simulink model "pneumatic04212025"  (R2024b)
settings: Solver=VariableStepAuto  StartTime=0.0  StopTime=20  RelTol=1e-3
values from neighbouring files (symbols this model uses):
  A1 = 3.1416e-04    (= 0.00031416)    [InitialParameter.m]    (also in pneumatic_code.m = 0.000314159265359)
  A2 = 2.6389e-04    (= 0.00026389)    [InitialParameter.m]    (also in pneumatic_code.m = 0.000263893782902)
  Ap = Ar    (= 5.02654824574e-05)    [pneumatic_code.m]
  b = 1    [InitialParameter.m]    (also in pneumatic_code.m = 0.0025)
  Beta = 50    [pneumatic_code.m]
  beta_s = 8*10^-3    (= 0.008)    [pneumatic_code.m]
  C1 = sqrt((k/R)*(2/(k+1))^((k+1)/(k-1)))    [pneumatic_code.m]
  C2 = sqrt((2*k)/(R*(k-1)))    [pneumatic_code.m]
  Cf = .25    (= 0.25)    [pneumatic_code.m]
  ep = 0.0024    [InitialParameter.m]    (also in pneumatic_code.m = 0.02)
  g1 = 9    [InitialParameter.m]    (also in pneumatic_code.m = 10)
  g2 = 4    [InitialParameter.m]    (also in pneumatic_code.m = 9)
  g3 = 18    [InitialParameter.m]    (also in pneumatic_code.m = 5)
  g4 = 0.32    [InitialParameter.m]    (also in pneumatic_code.m = 3)
  g5 = 3    [pneumatic_code.m]
  gamma1 = R*T*k    (= 118129.2)    [pneumatic_code.m]
  k = 1.4    [pneumatic_code.m]
  k1 = wc^4    (= 81450625)    [InitialParameter.m]    (also in pneumatic_code.m = 3620506.28125)
  k2 = 4*wc^3    (= 3429500)    [InitialParameter.m]    (also in pneumatic_code.m = 883050.3125)
  k3 = 6*wc^2    (= 54150)    [InitialParameter.m]    (also in pneumatic_code.m = 86151.25)
  k4 = 4*wc    (= 380)    [InitialParameter.m]    (also in pneumatic_code.m = 4202.5)
  k5 = 5*(wc)    (= 102.5)    [pneumatic_code.m]
  ke = 50    [pneumatic_code.m]
  ks = 7.5    [pneumatic_code.m]
  L = 0.15    [InitialParameter.m]    (also in pneumatic_code.m)
  M = 0.1    [InitialParameter.m]    (also in pneumatic_code.m)
  Ms = 0.5    [InitialParameter.m]    (also in pneumatic_code.m)
  nh = 4    [InitialParameter.m]    (also in pneumatic_code.m)
  Patm = 101352    [pneumatic_code.m]
  Pcr = (2/(k+1))^(k/(k-1))    (= 0.528281787717)    [pneumatic_code.m]
  Psum = 758423    [pneumatic_code.m]
  Pw = 0.0024    [InitialParameter.m]    (also in pneumatic_code.m = 0.0025)
  Rh = 0.0019    [InitialParameter.m]    (also in pneumatic_code.m)
  Rs = 13.5    [InitialParameter.m]    (also in pneumatic_code.m)
  T = 294    [pneumatic_code.m]
  Vinact = 1e-04    (= 0.0001)    [InitialParameter.m]    (also in pneumatic_code.m)
  WallForce = 1E12    (= 1000000000000)    [pneumatic_code.m]
  WallPose = 0.1    [pneumatic_code.m]
  Xinact = 1E-4    (= 0.0001)    [pneumatic_code.m]
undefined symbols (not defined in the file or in its folder): sigbuilder_block
settings Model: Creator=mandalia  LastModifiedBy=pangl

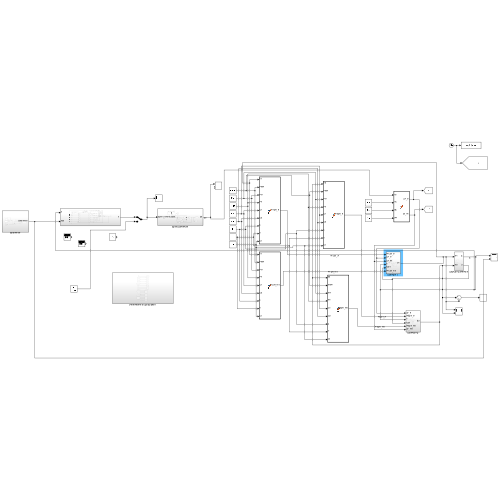
[thumbnail: Simulink's stored preview of the top-level diagram]
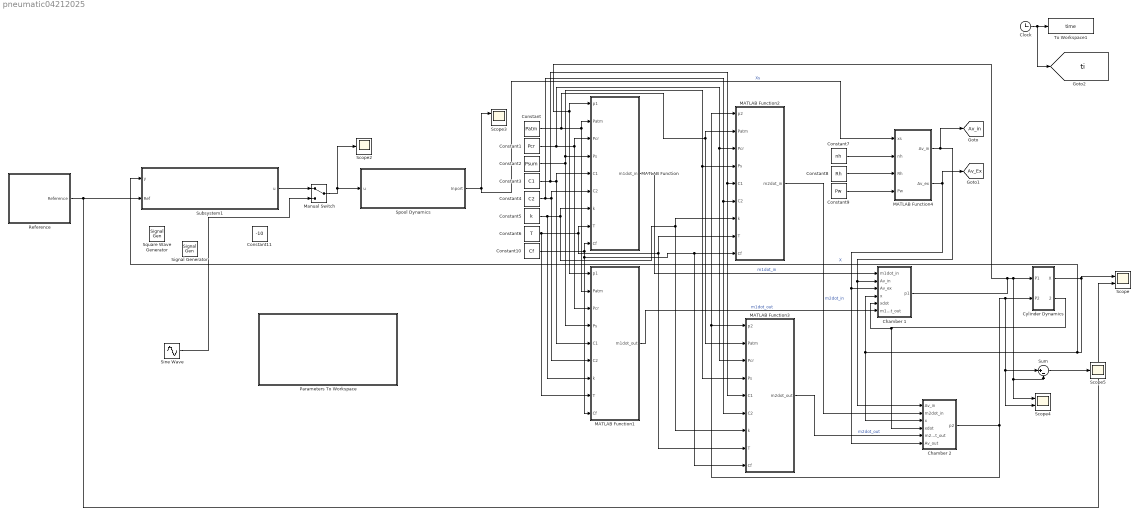
== system pneumatic04212025 ==
  "Chamber 1 " : Subsystem
  Chamber 2 : Subsystem
  Clock : Clock
  Constant : Constant  Value=Patm
  Constant1 : Constant  Value=Pcr
  Constant10 : Constant  Value=Cf
  Constant11 : Constant  Value=-10
  Constant2 : Constant  Value=Psum
  Constant3 : Constant  Value=C1
  Constant4 : Constant  Value=C2
  Constant5 : Constant  Value=k
  Constant6 : Constant  Value=T
  Constant7 : Constant  Value=nh
  Constant8 : Constant  Value=Rh
  Constant9 : Constant  Value=Pw
  Cylinder Dynamics : Subsystem
  MATLAB Function : MATLAB Function  TreatAsAtomicUnit=on
  MATLAB Function1 : MATLAB Function  TreatAsAtomicUnit=on
  MATLAB Function2 : MATLAB Function  TreatAsAtomicUnit=on
  MATLAB Function3 : MATLAB Function  TreatAsAtomicUnit=on
  MATLAB Function4 : MATLAB Function  TreatAsAtomicUnit=on
  Manual Switch : ManualSwitch
  Parameters To Workspace : Subsystem
  Reference : Subsystem
  Scope : Scope  NumInputPorts=2
  Scope2 : Scope
  Scope3 : Scope  NumInputPorts=2
  Scope4 : Scope  NumInputPorts=2
  Scope5 : Scope
  Signal Generator : SignalGenerator  Units=rad/sec
  Sine Wave : Sin  Amplitude=10  Frequency=120  SampleTime=0
  Spool Dynamics : Subsystem
  Square Wave Generator : SignalGenerator  WaveForm=square  Amplitude=4  Units=rad/sec
  Subsystem1 : Subsystem
  Sum : Sum  Inputs=|+-
  To Workspace1 : ToWorkspace  VariableName=time  SampleTime=-1
  tag scope: Av_Ex=global, Av_in=global, ti=global
  wires:
  Clock/1 -> [ti], To Workspace1/1
  Constant10/1 -> MATLAB Function3/9(Cf), MATLAB Function2/9(Cf), MATLAB Function1/9(Cf), MATLAB Function/9(Cf)
  Constant2/1 -> MATLAB Function3/4(Ps), MATLAB Function2/4(Ps), MATLAB Function/4(Ps), MATLAB Function1/4(Ps)
  Sum/1 -> Scope5/1
  Constant1/1 -> MATLAB Function3/3(Pcr), MATLAB Function2/3(Pcr), MATLAB Function1/3(Pcr), MATLAB Function/3(Pcr)
  Constant8/1 -> MATLAB Function4/3(Rh)
  Manual Switch/1 -> Scope2/1, Spool Dynamics/1(u)
  "Chamber 1 "/1(p1) -> MATLAB Function1/1(p1), MATLAB Function/1(p1), Sum/2, Scope4/1, Cylinder Dynamics/1(P1)
  Reference/1(Reference) -> Subsystem1/2(Ref), Scope/2
  Spool Dynamics/1(Inport) -> Scope3/1, MATLAB Function4/1(xs)  "Xs"
  Cylinder Dynamics/2(Out2) -> Chamber 2/4(xdot), "Chamber 1 "/5(xdot)
  Constant4/1 -> MATLAB Function3/6(C2), MATLAB Function2/6(C2), MATLAB Function1/6(C2), MATLAB Function/6(C2)
  MATLAB Function4/2(Av_ex) -> [Av_Ex], "Chamber 1 "/3(Av_ex), Chamber 2/6(Av_out)
  Constant5/1 -> MATLAB Function1/7(k), MATLAB Function3/7(k), MATLAB Function2/7(k), MATLAB Function/7(k)
  MATLAB Function2/1(m2dot_in) -> Chamber 2/2(m2dot_in)  "m2dot_in"
  Constant/1 -> MATLAB Function3/2(Patm), MATLAB Function2/2(Patm), MATLAB Function1/2(Patm), MATLAB Function/2(Patm)
  MATLAB Function3/1(m2dot_out) -> Chamber 2/5(m2dot_out)  "m2dot_out"
  MATLAB Function1/1(m1dot_out) -> "Chamber 1 "/6(m1dot_out)  "m1dot_out"
  Constant6/1 -> MATLAB Function3/8(T), MATLAB Function2/8(T), MATLAB Function/8(T), MATLAB Function1/8(T)
  MATLAB Function4/1(Av_in) -> [Av_in], "Chamber 1 "/2(Av_in), Chamber 2/1(Av_in)
  Constant3/1 -> MATLAB Function3/5(C1), MATLAB Function2/5(C1), MATLAB Function1/5(C1), MATLAB Function/5(C1)
  Cylinder Dynamics/1(X) -> Scope/1, Subsystem1/1(y), Chamber 2/3(x), "Chamber 1 "/4(x)  "X"
  Constant7/1 -> MATLAB Function4/2(nh)
  Chamber 2/1(p2) -> Sum/1, Scope4/2, Cylinder Dynamics/2(P2), MATLAB Function2/1(p2), MATLAB Function3/1(p2)
  Constant9/1 -> MATLAB Function4/4(Pw)
  MATLAB Function/1(m1dot_in) -> "Chamber 1 "/1(m1dot_in)  "m1dot_in"
  Subsystem1/1(u) -> Manual Switch/1
  Sine Wave/1 -> Manual Switch/2

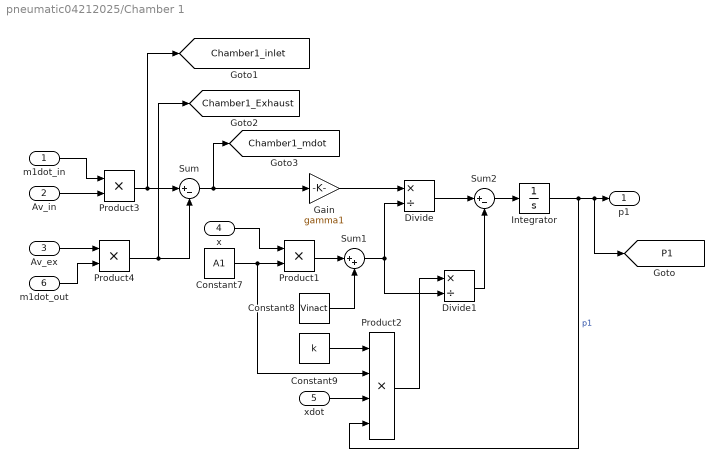
== system pneumatic04212025/Chamber 1  ==
  m1dot_in : Inport
  Av_in : Inport  Port=2
  Av_ex : Inport  Port=3
  x : Inport  Port=4
  xdot : Inport  Port=5
  m1dot_out : Inport  Port=6
  Constant7 : Constant  Value=A1
  Constant8 : Constant  Value=Vinact
  Constant9 : Constant  Value=k
  Divide : Product  Inputs=*/
  Divide1 : Product  Inputs=*/
  Gain : Gain  Gain=gamma1
  Integrator : Integrator  InitialCondition=Patm  LimitOutput=on  UpperSaturationLimit=Psum  LowerSaturationLimit=Patm
  Product1 : Product
  Product2 : Product  Inputs=4
  Product3 : Product
  Product4 : Product
  Sum : Sum  Inputs=|+-
  Sum1 : Sum  Inputs=|++
  Sum2 : Sum  Inputs=|+-
  p1 : Outport
  tag scope: Chamber1_Exhaust=global, Chamber1_inlet=global, Chamber1_mdot=global, P1=global
  wires:
  Divide/1 -> Sum2/1
  Constant8/1 -> Sum1/2
  Product1/1 -> Sum1/1
  Sum/1 -> [Chamber1_mdot], Gain/1
  Gain/1 -> Divide/1
  Constant7/1 -> Product1/2, Product2/2
  Divide1/1 -> Sum2/2
  Constant9/1 -> Product2/1
  Sum1/1 -> Divide1/2, Divide/2
  x/1 -> Product1/1
  Product2/1 -> Divide1/1
  Integrator/1 -> [P1], p1/1, Product2/4  "p1"
  Sum2/1 -> Integrator/1
  m1dot_in/1 -> Product3/1
  xdot/1 -> Product2/3
  Product4/1 -> [Chamber1_Exhaust], Sum/2
  Av_in/1 -> Product3/2
  Product3/1 -> [Chamber1_inlet], Sum/1
  m1dot_out/1 -> Product4/2
  Av_ex/1 -> Product4/1

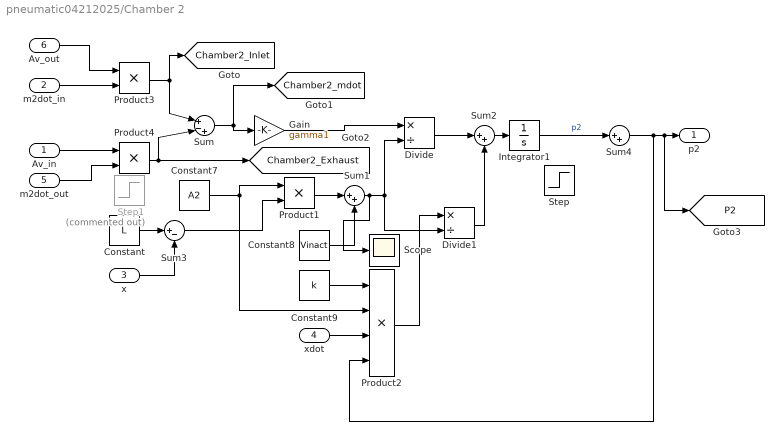
== system pneumatic04212025/Chamber 2 ==
  Av_in : Inport
  m2dot_in : Inport  Port=2
  x : Inport  Port=3
  xdot : Inport  Port=4
  m2dot_out : Inport  Port=5
  Av_out : Inport  Port=6
  Constant : Constant  Value=L
  Constant7 : Constant  Value=A2
  Constant8 : Constant  Value=Vinact
  Constant9 : Constant  Value=k
  Divide : Product  Inputs=*/
  Divide1 : Product  Inputs=*/
  Gain : Gain  Gain=gamma1
  Integrator1 : Integrator  InitialCondition=Patm  LimitOutput=on  UpperSaturationLimit=Psum  LowerSaturationLimit=Patm
  Product1 : Product
  Product2 : Product  Inputs=4
  Product3 : Product
  Product4 : Product
  Scope : Scope
  Step : Step  Time=5  After=-10*10^3  SampleTime=0
  Step1 : Step  Commented=on  Time=5  After=-1*10^-3  SampleTime=0
  Sum : Sum  Inputs=|+-+
  Sum1 : Sum  Inputs=|++
  Sum2 : Sum  Inputs=|++
  Sum3 : Sum  Inputs=|+-
  Sum4 : Sum  Inputs=|++
  p2 : Outport
  tag scope: Chamber2_Exhaust=global, Chamber2_Inlet=global, Chamber2_mdot=global, P2=global
  wires:
  m2dot_out/1 -> Product4/2
  xdot/1 -> Product2/3
  Sum2/1 -> Integrator1/1
  Integrator1/1 -> Sum4/1  "p2"
  Product2/1 -> Divide1/1
  Sum1/1 -> Scope/1, Divide/2, Divide1/2
  Constant9/1 -> Product2/1
  Divide1/1 -> Sum2/2
  Constant7/1 -> Product2/2, Product1/1
  Gain/1 -> Divide/1
  Sum/1 -> Gain/1, [Chamber2_mdot]
  Product1/1 -> Sum1/1
  Constant8/1 -> Sum1/2
  Divide/1 -> Sum2/1
  x/1 -> Sum3/2
  Constant/1 -> Sum3/1
  Sum3/1 -> Product1/2
  Av_in/1 -> Product4/1
  m2dot_in/1 -> Product3/2
  Product3/1 -> [Chamber2_Inlet], Sum/1
  Av_out/1 -> Product3/1
  Product4/1 -> [Chamber2_Exhaust], Sum/2
  Sum4/1 -> [P2], p2/1, Product2/4

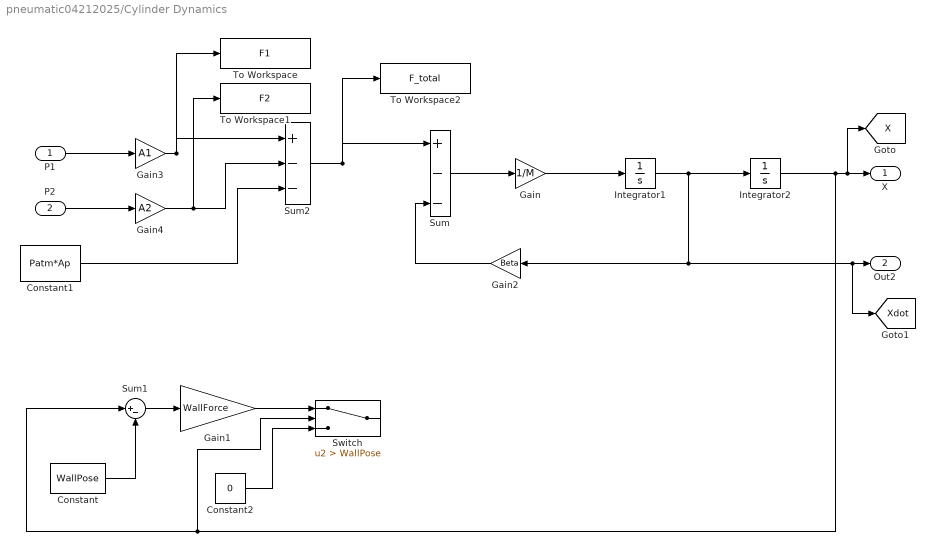
== system pneumatic04212025/Cylinder Dynamics ==
  P1 : Inport
  P2 : Inport  Port=2
  Constant : Constant  Value=WallPose
  Constant1 : Constant  Value=Patm*Ap
  Constant2 : Constant  Value=0
  Gain : Gain  Gain=1/M
  Gain1 : Gain  Gain=WallForce
  Gain2 : Gain  Gain=Beta
  Gain3 : Gain  Gain=A1
  Gain4 : Gain  Gain=A2
  Integrator1 : Integrator
  Integrator2 : Integrator  InitialCondition=Xinact  LimitOutput=on  UpperSaturationLimit=L  LowerSaturationLimit=Xinact
  Sum : Sum  Inputs=|+--
  Sum1 : Sum  Inputs=|+-
  Sum2 : Sum  Inputs=|+--
  Switch : Switch  Criteria=u2 > Threshold  Threshold=WallPose  SaturateOnIntegerOverflow=off  InputSameDT=off
  To Workspace : ToWorkspace  VariableName=F1  SampleTime=-1
  To Workspace1 : ToWorkspace  VariableName=F2  SampleTime=-1
  To Workspace2 : ToWorkspace  VariableName=F_total  SampleTime=-1
  X : Outport
  Out2 : Outport  Port=2
  tag scope: X=global, Xdot=global
  wires:
  Integrator2/1 -> Switch/2, Sum1/1, [X], X/1
  Integrator1/1 -> Integrator2/1, [Xdot], Out2/1, Gain2/1
  Gain4/1 -> To Workspace1/1, Sum2/2
  Gain2/1 -> Sum/3
  Gain/1 -> Integrator1/1
  Sum/1 -> Gain/1
  Sum2/1 -> To Workspace2/1, Sum/1
  P2/1 -> Gain4/1
  P1/1 -> Gain3/1
  Gain3/1 -> To Workspace/1, Sum2/1
  Constant1/1 -> Sum2/3
  Constant/1 -> Sum1/2
  Sum1/1 -> Gain1/1
  Gain1/1 -> Switch/1
  Constant2/1 -> Switch/3

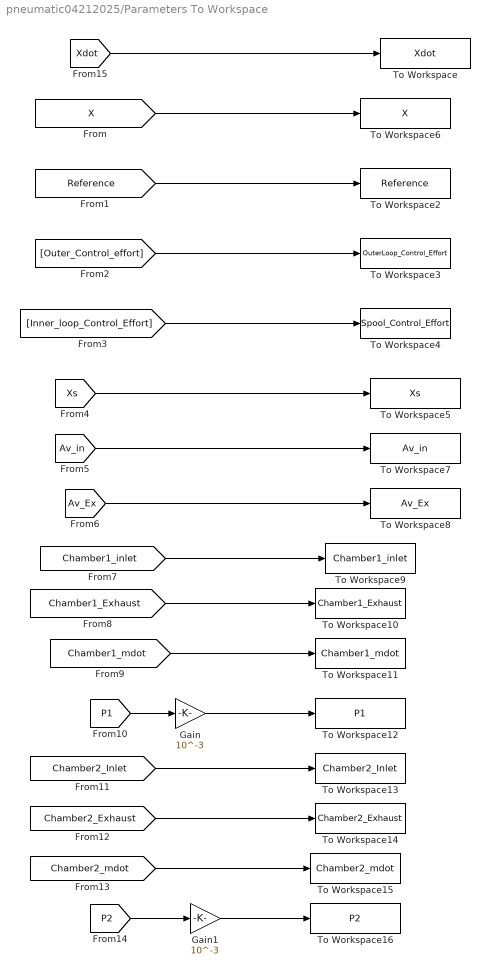
== system pneumatic04212025/Parameters To Workspace ==
  Gain : Gain  Gain=10^-3
  Gain1 : Gain  Gain=10^-3
  To Workspace : ToWorkspace  VariableName=Xdot  SampleTime=-1
  To Workspace10 : ToWorkspace  VariableName=Chamber1_Exhaust  SampleTime=-1
  To Workspace11 : ToWorkspace  VariableName=Chamber1_mdot  SampleTime=-1
  To Workspace12 : ToWorkspace  VariableName=P1  SampleTime=-1
  To Workspace13 : ToWorkspace  VariableName=Chamber2_Inlet  SampleTime=-1
  To Workspace14 : ToWorkspace  VariableName=Chamber2_Exhaust  SampleTime=-1
  To Workspace15 : ToWorkspace  VariableName=Chamber2_mdot  SampleTime=-1
  To Workspace16 : ToWorkspace  VariableName=P2  SampleTime=-1
  To Workspace2 : ToWorkspace  VariableName=Reference  SampleTime=-1
  To Workspace3 : ToWorkspace  VariableName=OuterLoop_Control_Effort  SampleTime=-1
  To Workspace4 : ToWorkspace  VariableName=Spool_Control_Effort  SampleTime=-1
  To Workspace5 : ToWorkspace  VariableName=Xs  SampleTime=-1
  To Workspace6 : ToWorkspace  VariableName=X  SampleTime=-1
  To Workspace7 : ToWorkspace  VariableName=Av_in  SampleTime=-1
  To Workspace8 : ToWorkspace  VariableName=Av_Ex  SampleTime=-1
  To Workspace9 : ToWorkspace  VariableName=Chamber1_inlet  SampleTime=-1
  wires:
  [Reference] -> To Workspace2/1
  [Xs] -> To Workspace5/1
  [Av_Ex] -> To Workspace8/1
  [Chamber1_Exhaust] -> To Workspace10/1
  [X] -> To Workspace6/1
  [Outer_Control_effort] -> To Workspace3/1
  [Chamber2_Exhaust] -> To Workspace14/1
  [Inner_loop_Control_Effort] -> To Workspace4/1
  [P2] -> Gain1/1
  [Av_in] -> To Workspace7/1
  [P1] -> Gain/1
  [Chamber2_mdot] -> To Workspace15/1
  [Chamber2_Inlet] -> To Workspace13/1
  [Chamber1_mdot] -> To Workspace11/1
  [Chamber1_inlet] -> To Workspace9/1
  [Xdot] -> To Workspace/1
  Gain/1 -> To Workspace12/1
  Gain1/1 -> To Workspace16/1

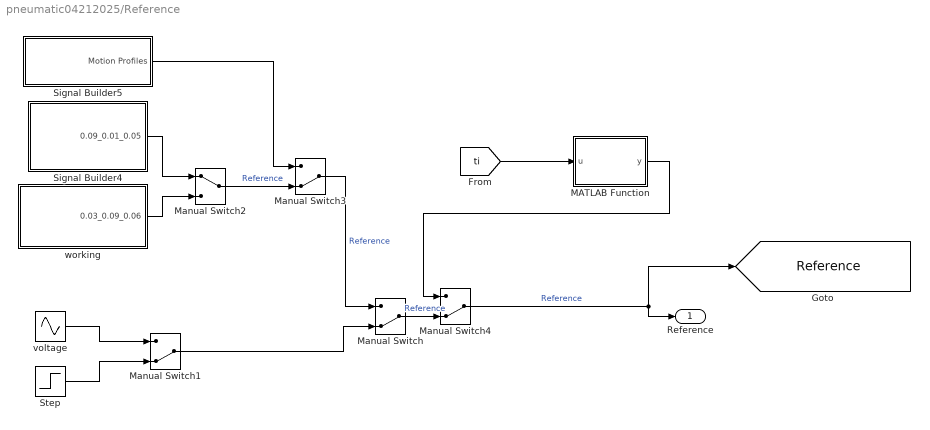
== system pneumatic04212025/Reference ==
  MATLAB Function : MATLAB Function  TreatAsAtomicUnit=on
  Manual Switch{,1,3..4} (4 alike) : ManualSwitch  CurrentSetting=0
  Manual Switch2 : ManualSwitch
  Signal Builder4 : Subsystem  Tag=STV Subsys  LoadFcn=sigbuilder_block('load');  StartFcn=sigbuilder_block('start');  StopFcn=sigbuilder_block('stop');  ClipboardFcn=sigbuilder_block('clipboard');  mask(Sigbuilder block){tuvar=[0:10]}
      mask help: Simulink:masks:SigbuilderBlock_MD
      mask init:
      | if ~strcmp(get_param(bdroot(gcbh),'SimulationStatus'),'stopped') tuvar = sigbuilder_block('maskInit'); end
      settings: CopyFcn=sigbuilder_block('copy');  DeleteFcn=sigbuilder_block('delete');  ModelCloseFcn=sigbuilder_block('modelClose');  PreSaveFcn=sigbuilder_block('preSave');  PauseFcn=sigbuilder_block('pause');  ContinueFcn=sigbuilder_block('continue');  NameChangeFcn=sigbuilder_block('namechange');  OpenFcn=sigbuilder_block('open',[5.4 84 1141.2 548 ]);  CloseFcn=sigbuilder_block('close');
      mask Display: plot(0, 0, 100, 100,[2, 2, 32, 32, 2], [68, 8, 8, 68, 68],[32, 2], [38, 38], [32, 19, 2],[53, 60, 44], [32, 17, 17, 2],[16, 16, 31, 31]);txt = getActiveGroup(gcbh);text(2, 100, txt,'verticalAlignment', 'top');
  Signal Builder5 : Subsystem  Tag=STV Subsys  LoadFcn=sigbuilder_block('load');  StartFcn=sigbuilder_block('start');  StopFcn=sigbuilder_block('stop');  ClipboardFcn=sigbuilder_block('clipboard');  mask(Sigbuilder block){tuvar=[0:10]}
      mask help: Simulink:masks:SigbuilderBlock_MD
      mask init:
      | if ~strcmp(get_param(bdroot(gcbh),'SimulationStatus'),'stopped') tuvar = sigbuilder_block('maskInit'); end
      settings: CopyFcn=sigbuilder_block('copy');  DeleteFcn=sigbuilder_block('delete');  ModelCloseFcn=sigbuilder_block('modelClose');  PreSaveFcn=sigbuilder_block('preSave');  PauseFcn=sigbuilder_block('pause');  ContinueFcn=sigbuilder_block('continue');  NameChangeFcn=sigbuilder_block('namechange');  OpenFcn=sigbuilder_block('open',[5.4 84 1141.2 548 ]);  CloseFcn=sigbuilder_block('close');
      mask Display: plot(0, 0, 100, 100,[2, 2, 32, 32, 2], [68, 8, 8, 68, 68],[32, 2], [38, 38], [32, 19, 2],[53, 60, 44], [32, 17, 17, 2],[16, 16, 31, 31]);txt = getActiveGroup(gcbh);text(2, 100, txt,'verticalAlignment', 'top');
  Step : Step  Time=0  Before=Xinact  After=0.09  SampleTime=0
  voltage : Sin  Amplitude=0.02  Bias=0.06  Frequency=(2*pi)/20  SampleTime=0
  working : Subsystem  Tag=STV Subsys  LoadFcn=sigbuilder_block('load');  StartFcn=sigbuilder_block('start');  StopFcn=sigbuilder_block('stop');  ClipboardFcn=sigbuilder_block('clipboard');  mask(Sigbuilder block){tuvar=[0:10]}
      mask help: Simulink:masks:SigbuilderBlock_MD
      mask init:
      | if ~strcmp(get_param(bdroot(gcbh),'SimulationStatus'),'stopped') tuvar = sigbuilder_block('maskInit'); end
      settings: CopyFcn=sigbuilder_block('copy');  DeleteFcn=sigbuilder_block('delete');  ModelCloseFcn=sigbuilder_block('modelClose');  PreSaveFcn=sigbuilder_block('preSave');  PauseFcn=sigbuilder_block('pause');  ContinueFcn=sigbuilder_block('continue');  NameChangeFcn=sigbuilder_block('namechange');  OpenFcn=sigbuilder_block('open',[5.4 84 1141.2 548 ]);  CloseFcn=sigbuilder_block('close');
      mask Display: plot(0, 0, 100, 100,[2, 2, 32, 32, 2], [68, 8, 8, 68, 68],[32, 2], [38, 38], [32, 19, 2],[53, 60, 44], [32, 17, 17, 2],[16, 16, 31, 31]);txt = getActiveGroup(gcbh);text(2, 100, txt,'verticalAlignment', 'top');
  Reference : Outport
  tag scope: Reference=global
  wires:
  Step/1 -> Manual Switch1/2
  voltage/1 -> Manual Switch1/1
  Manual Switch2/1 -> Manual Switch3/2  "Reference"
  Manual Switch3/1 -> Manual Switch/1  "Reference"
  Manual Switch4/1 -> Reference/1, [Reference]  "Reference"
  Signal Builder4/1(0.09_0.01_0.05) -> Manual Switch2/1
  working/1(0.03_0.09_0.06) -> Manual Switch2/2
  Manual Switch1/1 -> Manual Switch/2
  Signal Builder5/1(Motion Profiles) -> Manual Switch3/1
  [ti] -> MATLAB Function/1(u)
  Manual Switch/1 -> Manual Switch4/2  "Reference"
  MATLAB Function/1(y) -> Manual Switch4/1

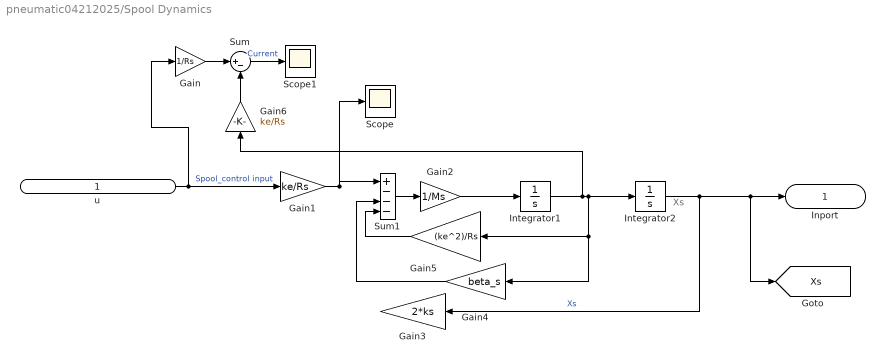
== system pneumatic04212025/Spool Dynamics ==
  note: Xs
  u : Inport
  Gain : Gain  Gain=1/Rs
  Gain1 : Gain  Gain=ke/Rs
  Gain2 : Gain  Gain=1/Ms
  Gain3 : Gain  Gain=2*ks
  Gain4 : Gain  Gain=beta_s
  Gain5 : Gain  Gain=(ke^2)/Rs
  Gain6 : Gain  Gain=ke/Rs
  Integrator1 : Integrator
  Integrator2 : Integrator  LimitOutput=on  UpperSaturationLimit=1.1*1e-3  LowerSaturationLimit=-1.1*1e-3
  Scope : Scope
  Scope1 : Scope
  Sum : Sum  Inputs=|+-
  Sum1 : Sum  Inputs=|+---
  Inport : Outport
  tag scope: Xs=global
  wires:
  Gain4/1 -> Sum1/3
  Integrator1/1 -> Gain6/1, Gain5/1, Gain4/1, Integrator2/1
  Gain5/1 -> Sum1/4
  Sum1/1 -> Gain2/1
  Gain1/1 -> Scope/1, Sum1/1
  Gain2/1 -> Integrator1/1
  Integrator2/1 -> [Xs], Inport/1, Gain3/1  "Xs"
  u/1 -> Gain/1, Gain1/1  "Spool_control input"
  Gain/1 -> Sum/1
  Gain6/1 -> Sum/2
  Sum/1 -> Scope1/1  "Current"

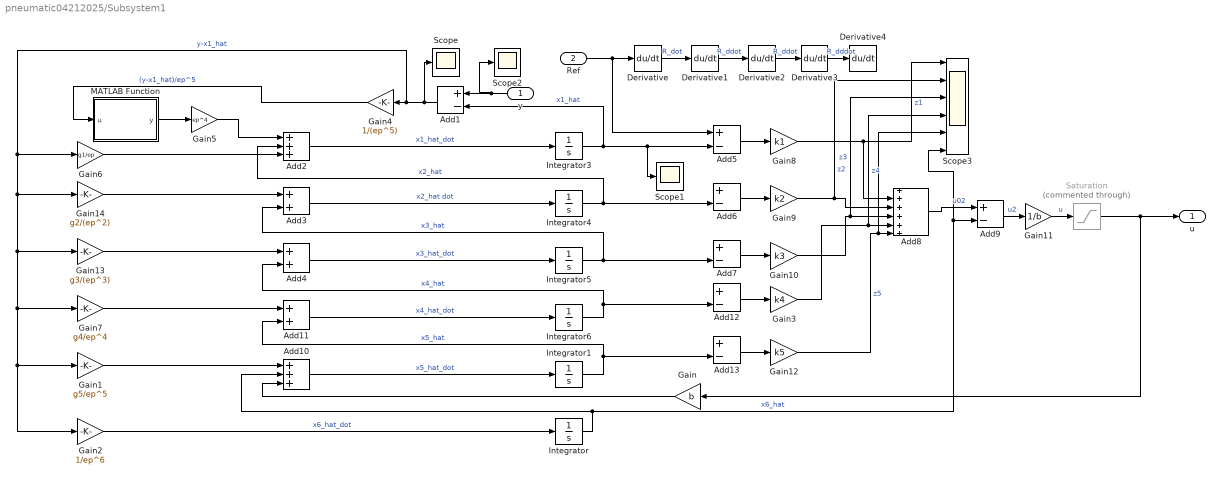
== system pneumatic04212025/Subsystem1 ==
  y : Inport
  Ref : Inport  Port=2
  Add{1,5..7,9,12..13} (7 alike) : Sum  Inputs=+-
  Add10 : Sum  Inputs=+++
  Add11 : Sum
  Add2 : Sum  Inputs=+++
  Add3 : Sum
  Add4 : Sum
  Add8 : Sum  Inputs=++++++
  Derivative{,1..4} (5 alike) : Derivative
  Gain : Gain  Gain=b
  Gain1 : Gain  Gain=g5/ep^5
  Gain10 : Gain  Gain=k3
  Gain11 : Gain  Gain=1/b
  Gain12 : Gain  Gain=k5
  Gain13 : Gain  Gain=g3/(ep^3)
  Gain14 : Gain  Gain=g2/(ep^2)
  Gain2 : Gain  Gain=1/ep^6
  Gain3 : Gain  Gain=k4
  Gain4 : Gain  Gain=1/(ep^5)
  Gain5 : Gain  Gain=ep^4
  Gain6 : Gain  Gain=g1/ep
  Gain7 : Gain  Gain=g4/ep^4
  Gain8 : Gain  Gain=k1
  Gain9 : Gain  Gain=k2
  Integrator{,1,4..6} (5 alike) : Integrator
  Integrator3 : Integrator  UpperSaturationLimit=0.15  LowerSaturationLimit=1e-4
  MATLAB Function : MATLAB Function  TreatAsAtomicUnit=on
  Saturation : Saturate  Commented=through  UpperLimit=10  LowerLimit=-10
  Scope : Scope
  Scope1 : Scope
  Scope2 : Scope
  Scope3 : Scope  NumInputPorts=6
  u : Outport
  wires:
  Add12/1 -> Gain3/1
  Add6/1 -> Gain9/1
  Derivative1/1 -> Derivative2/1  "R_ddot"
  Integrator3/1 -> Add1/2, Scope1/1, Add5/2  "x1_hat"
  Integrator4/1 -> Add6/2, Add2/2  "x2_hat"
  Integrator1/1 -> Add13/2, Add11/2  "x5_hat"
  Derivative/1 -> Derivative1/1  "R_dot"
  Gain12/1 -> Scope3/5, Add8/6  "z5"
  Add13/1 -> Gain12/1
  Gain1/1 -> Add10/1
  Integrator/1 -> Scope3/6, Add9/2, Add10/2  "x6_hat"
  Gain/1 -> Add10/3
  Gain7/1 -> Add11/1
  Gain5/1 -> Add2/1
  Gain11/1 -> Saturation/1  "u"
  Gain14/1 -> Add3/1
  Add11/1 -> Integrator6/1  "x4_hat_dot"
  Ref/1 -> Add5/1, Derivative/1
  Gain10/1 -> Scope3/3, Add8/4  "z3"
  Add4/1 -> Integrator5/1  "x3_hat_dot"
  Add1/1 -> Scope/1, Gain6/1, Gain2/1, Gain1/1, Gain7/1, Gain13/1, Gain14/1, Gain4/1  "y-x1_hat"
  Gain3/1 -> Scope3/4, Add8/5  "z4"
  Gain6/1 -> Add2/3
  Add5/1 -> Gain8/1
  Integrator5/1 -> Add7/2, Add3/2  "x3_hat"
  Add7/1 -> Gain10/1
  MATLAB Function/1(y) -> Gain5/1
  Integrator6/1 -> Add12/2, Add4/2  "x4_hat"
  Add9/1 -> Gain11/1  "u2"
  Gain8/1 -> Add8/2, Scope3/1  "z1"
  Derivative2/1 -> Derivative3/1  "R_ddot"
  Add3/1 -> Integrator4/1  "x2_hat dot"
  Add2/1 -> Integrator3/1  "x1_hat_dot"
  y/1 -> Scope2/1, Add1/1
  Gain9/1 -> Scope3/2, Add8/3  "z2"
  Gain4/1 -> MATLAB Function/1(u)  "(y-x1_hat)/ep^5"
  Gain13/1 -> Add4/1
  Add10/1 -> Integrator1/1  "x5_hat_dot"
  Gain2/1 -> Integrator/1  "x6_hat_dot"
  Derivative3/1 -> Derivative4/1  "R_dddot"
  Add8/1 -> Add9/1  "u02"
  Saturation/1 -> Gain/1, u/1

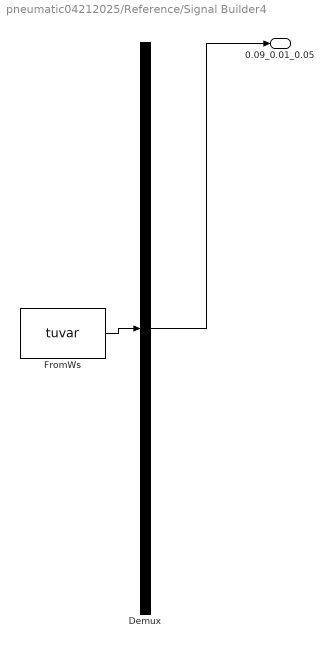
== system pneumatic04212025/Reference/Signal Builder4 ==
  Demux : Demux  Tag=STV Demux  Outputs=1
      settings: DisplayOption=none
  FromWs : FromWorkspace  Tag=STV FromWs  VariableName=tuvar
      SigBuilderData=|
      | common.afterFinalStr = 'Extrapolate'
      | common.sampleTime = 0
      | dataSet.timeRange = [0 6]
      | dataSet.name = 'Group 1'
      | sbobj.Groups.Name = 'Group 1'
      | sbobj.Groups.Signals.Name = '0.09_0.01_0.05'
      | sbobj.Groups.Signals.XData = [0 2 2 4 4 6]
      | sbobj.Groups.Signals.YData = [0.09 0.09 0.01 0.01 0.05 0.05]
      | sbobj.Groups.TimeRange = [0 6]
  0.09_0.01_0.05 : Outport  Tag=STV Outport
  wires:
  Demux/1 -> 0.09_0.01_0.05/1
  FromWs/1 -> Demux/1

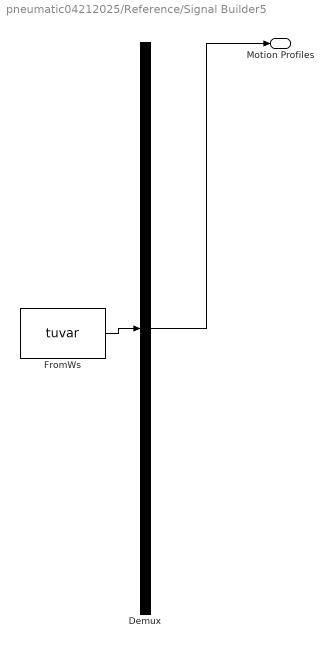
== system pneumatic04212025/Reference/Signal Builder5 ==
  Demux : Demux  Tag=STV Demux  Outputs=1
      settings: DisplayOption=none
  FromWs : FromWorkspace  Tag=STV FromWs  VariableName=tuvar
      SigBuilderData=|
      | common.afterFinalStr = 'Extrapolate'
      | common.sampleTime = 0
      | dataSet.timeRange = [0 10]
      | dataSet.name = 'Group 1'
      | sbobj.Groups.Name = 'Group 1'
      | sbobj.Groups.Signals.Name = 'Motion Profiles'
      | sbobj.Groups.Signals.XData = [0 0.4 1 1.4 2 3.6 4 5.4 6 8 8.6 10]
      | sbobj.Groups.Signals.YData = [0.02 0.02 0.02 0.09 0.09 0.0898 0.02 0.02 0.06 0.06 0.0196 0.02]
  Motion Profiles : Outport  Tag=STV Outport
  wires:
  Demux/1 -> Motion Profiles/1
  FromWs/1 -> Demux/1

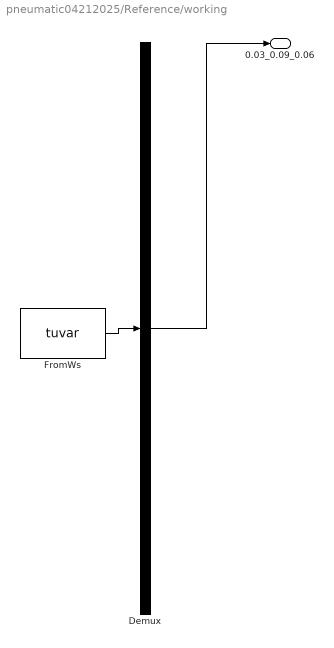
== system pneumatic04212025/Reference/working ==
  Demux : Demux  Tag=STV Demux  Outputs=1
      settings: DisplayOption=none
  FromWs : FromWorkspace  Tag=STV FromWs  VariableName=tuvar
      SigBuilderData=|
      | common.afterFinalStr = 'Extrapolate'
      | common.sampleTime = 0
      | dataSet.timeRange = [0 5]
      | dataSet.name = 'Group 1'
      | sbobj.Groups.Name = 'Group 1'
      | sbobj.Groups.Signals.Name = '0.03_0.09_0.06'
      | sbobj.Groups.Signals.XData = [0 2 2 4.005 4.005 5]
      | sbobj.Groups.Signals.YData = [0.03 0.03 0.09 0.09 0.06 0.06]
      | sbobj.Groups.TimeRange = [0 5]
  0.03_0.09_0.06 : Outport  Tag=STV Outport
  wires:
  Demux/1 -> 0.03_0.09_0.06/1
  FromWs/1 -> Demux/1

== matlab function pneumatic04212025/MATLAB Function1 ==
  data: p1 input; m1dot_out output; Patm input; Pcr input; Ps input; C1 input; C2 input; k input; T input; Cf input
function m1dot_out = fcn(p1,Patm,Pcr,Ps,C1,C2,k,T,Cf)
if (p1<Patm)
    p1=Patm;
elseif (p1>Ps)
    p1=Ps;
end
pu=p1;
pd=Patm;
Pratio=pd/pu;
if(Pratio <= Pcr && Pratio > 0)
    m1dot_out = Cf*C1*pu/sqrt(T);
elseif (Pratio > Pcr)
    m1dot_out = Cf*C2*pu/sqrt(T)*(pd/pu)^(1/k)*sqrt(1-(pd/pu)^((k-1)/k));
else
    m1dot_out = 0;
end

== matlab function pneumatic04212025/MATLAB Function ==
  data: p1 input; m1dot_in output; Patm input; Pcr input; Ps input; C1 input; C2 input; k input; T input; Cf input
function m1dot_in = fcn(p1,Patm,Pcr,Ps,C1,C2,k,T,Cf)
if (p1<Patm)
    p1=Patm;
elseif (p1>Ps)
    p1=Ps;
end
pu=Ps;
pd=p1;
Pratio=pd/pu;
if(Pratio <= Pcr && Pratio > 0)
    m1dot_in = Cf*C1*pu/sqrt(T);
elseif (Pratio > Pcr)
    m1dot_in = Cf*C2*pu/sqrt(T)*(pd/pu)^(1/k)*sqrt(1-(pd/pu)^((k-1)/k));
else
    m1dot_in = 0;
end

== matlab function pneumatic04212025/MATLAB Function2 ==
  data: p2 input; m2dot_in output; Patm input; Pcr input; Ps input; C1 input; C2 input; k input; T input; Cf input
function m2dot_in = fcn(p2,Patm,Pcr,Ps,C1,C2,k,T,Cf)
if (p2<Patm)
    p2=Patm;
elseif (p2>Ps)
    p2=Ps;
end
pu=Ps;
pd=p2;
Pratio=pd/pu;
if(Pratio <= Pcr && Pratio > 0)
    m2dot_in = Cf*C1*pu/sqrt(T);
elseif (Pratio > Pcr)
    m2dot_in = Cf*C2*pu/sqrt(T)*(pd/pu)^(1/k)*sqrt(1-(pd/pu)^((k-1)/k));
else
    m2dot_in = 0;
end

== matlab function pneumatic04212025/MATLAB Function3 ==
  data: p2 input; m2dot_out output; Patm input; Pcr input; Ps input; C1 input; C2 input; k input; T input; Cf input
function m2dot_out = fcn(p2,Patm,Pcr,Ps,C1,C2,k,T,Cf)
if (p2<Patm)
    p2=Patm;
elseif (p2>Ps)
    p2=Ps;
end
pu=p2;
pd=Patm;
Pratio=pd/pu;
if(Pratio <= Pcr && Pratio > 0)
    m2dot_out = Cf*C1*pu/sqrt(T);
elseif (Pratio > Pcr)
    m2dot_out = Cf*C2*pu/sqrt(T)*(pd/pu)^(1/k)*sqrt(1-(pd/pu)^((k-1)/k));
else
    m2dot_out = 0;
end

== matlab function pneumatic04212025/MATLAB Function4 ==
  data: xs input; Av_in output; nh input; Rh input; Pw input; Av_ex output
function [Av_in,Av_ex] = fcn(xs,nh,Rh,Pw)

if (xs <= (Pw-Rh))
    Av_in=0;
elseif (xs >= (Pw+Rh))
    Av_in=pi*nh*Rh^2;
else
    temp=sqrt((Rh-Pw+abs(xs))/(Rh+Pw-abs(xs)));
    Av_in=nh*((2*Rh*Rh*atan(temp))-((Pw-xs)*(sqrt((Rh^2)-(Pw-xs)^2))));
end
Xs=abs(xs);

if (xs <= (-Pw-Rh))
    Av_ex=pi*nh*Rh^2;
elseif (xs >= (Rh-Pw))
    Av_ex=0;
else
    temp1=sqrt((Rh-Pw+Xs)/(Rh+Pw-Xs));
    Av_ex=nh*((2*Rh*Rh*atan(temp1))-((Pw-Xs)*(sqrt((Rh^2)-(Pw-Xs)^2))));
end

== matlab function pneumatic04212025/Reference/MATLAB Function ==
  data: u input; y output
function y = fcn(u)

    y=1/(1+exp(-2*(u-0.5)));

== matlab function pneumatic04212025/Subsystem1/MATLAB Function ==
  data: u input; y output
function y = fcn(u)
y = 0;
if u <= -pi/2
    y = -(1/(4*pi));
elseif u <= pi/2 && u >= -pi/2
    y = sin(u)/(4*pi);
elseif u >=pi/2
    y = 1/(4*pi);
end
